simulink model "AERO421_FP6"  (R2024b)
settings: Solver=FixedStepAuto  StartTime=0.0  StopTime=tspan  FixedStep=5  RelTol=1e-5
values from neighbouring files (symbols this model uses):
  E_b_ECI_0 = C2EulerAngles(C_b_ECI_0)    [AERO421_FP6_RJFSR.m]    (also in stefansOldCode.m)
  I_s = diag([1.2, 1.2, 1.2])    [AERO421_FP6_RJFSR.m]    (also in stefansOldCode.m = diag([0.6, 0.6 ,1.2]))
  J = J + I_w1 + I_w2 + I_w3    [AERO421_FP6_RJFSR.m]    (also in stefansOldCode.m = J + I_s)
  Kd = J*eye(3)*2*zeta*wn    [AERO421_FP6_RJFSR.m]    (also in stefansOldCode.m)
  Kp = 2*J*eye(3)*wn^2    [AERO421_FP6_RJFSR.m]    (also in stefansOldCode.m)
  q_b_ECI_0 = rotm2quat(C_b_ECI_0)    [AERO421_FP6_RJFSR.m]    (also in stefansOldCode.m)
  w_b_ECI_0 = [0.001; -0.001; 0.002]    [AERO421_FP6_RJFSR.m]    (also in stefansOldCode.m)
undefined symbols (not defined in the file or in its folder): r_ECI_0, v_ECI_0
libraries: aerolibutil x1
settings Model: Creator=emehiel  LastModifiedBy=rosha
settings SolverCC: AlgebraicLoopSolver=TrustRegion
settings DebuggingCC: UnconnectedInputMsg=warning  UnconnectedOutputMsg=warning  UnconnectedLineMsg=warning
settings ModelReferenceCC: EnableRefExpFcnMdlSchedulingChecks=on
settings RTWCC: GPUComputeCapability=3.5

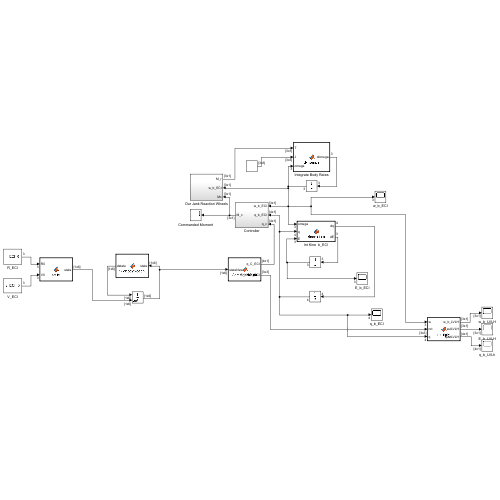
[thumbnail: Simulink's stored preview of the top-level diagram]
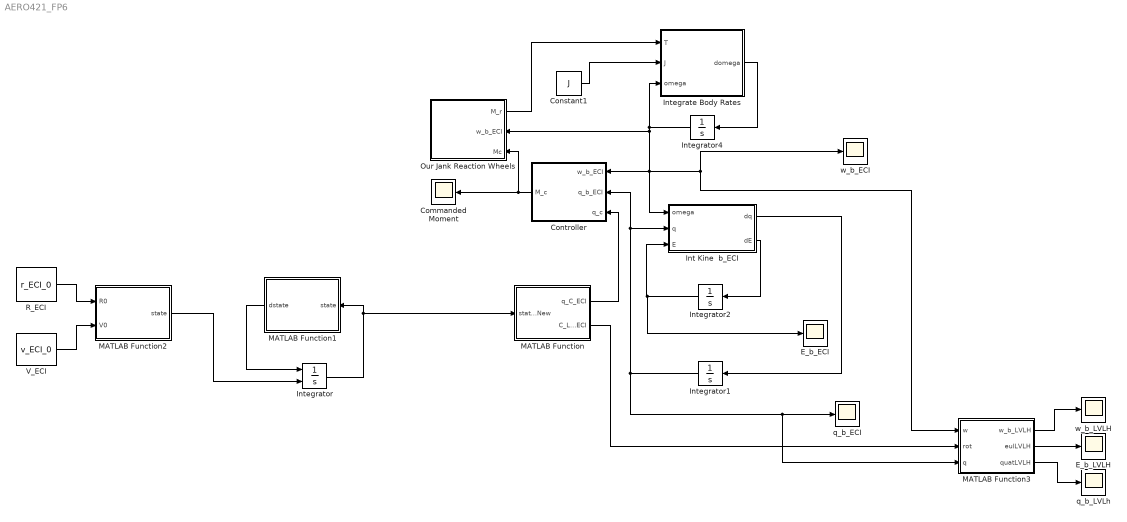
== system AERO421_FP6 ==
  Commanded Moment : Scope
  Constant1 : Constant  Value=J
  Controller : Subsystem
  E_b_ECI : Scope
  E_b_LVLH : Scope
  Int Kine  b_ECI : MATLAB Function  TreatAsAtomicUnit=on
  Integrate Body Rates : MATLAB Function  TreatAsAtomicUnit=on
  Integrator : Integrator  InitialConditionSource=external
  Integrator1 : Integrator  InitialCondition=q_b_ECI_0
  Integrator2 : Integrator  InitialCondition=E_b_ECI_0
  Integrator4 : Integrator  InitialCondition=w_b_ECI_0
  MATLAB Function : MATLAB Function  TreatAsAtomicUnit=on
  MATLAB Function1 : MATLAB Function  TreatAsAtomicUnit=on
  MATLAB Function2 : MATLAB Function  TreatAsAtomicUnit=on
  MATLAB Function3 : MATLAB Function  TreatAsAtomicUnit=on
  Our Jank Reaction Wheels : Subsystem
      settings: PortSchema="{\"entries\":[{\"content\":{\"sides\":[{\"content\":{\"connectorIds\":[\"Out1\",\"In1\",\"In2\"]},\"type\":\"ConnectorPlacement.EquallySpacedRectSide\",\"uuid\":\"c07e65a8-3a09-4163-ab9e-2228d2e52ec5\"},{\"content\":{\"side\":\"RIGHT\"},\"type\":\"ConnectorPlacement.EquallySpacedRectSide\",\"uuid\":\"64fc0568-6df4-40c5-97b1-a675a03b9b7b\"},{\"content\":{\"side\":\"TOP\"},\"type\":\"ConnectorPlacement.EquallySpacedRectSide\",\"uuid\":\"6ced51b5-350f-46bd-bff5-546870cdfb70\"}]},\"type\":\"ConnectorPlacement.EquallySpacedConnector\",\"uuid\":\"a6912720-308f-478a-9475-f02870833daa\"}],\"packageUris\":[\"http://schema.mathworks.com/mf0/Connector/R2020b\"],\"version\":\"1.0\"}"
  R_ECI : Constant  Value=r_ECI_0
  V_ECI : Constant  Value=v_ECI_0
  q_b_ECI : Scope
  q_b_LVLh : Scope
  w_b_ECI : Scope
  w_b_LVLH : Scope
  wires:
  Controller/1(M_c) -> Commanded Moment/1, Our Jank Reaction Wheels/2(Mc)
  Constant1/1 -> Integrate Body Rates/2(J)
  Integrate Body Rates/1(domega) -> Integrator4/1
  Integrator4/1 -> Our Jank Reaction Wheels/1(w_b_ECI), MATLAB Function3/1(w), w_b_ECI/1, Int Kine  b_ECI/1(omega), Controller/1(w_b_ECI), Integrate Body Rates/3(omega)
  Integrator2/1 -> E_b_ECI/1, Int Kine  b_ECI/3(E)
  Integrator1/1 -> Controller/2(q_b_ECI), Int Kine  b_ECI/2(q), MATLAB Function3/3(q), q_b_ECI/1
  Int Kine  b_ECI/2(dE) -> Integrator2/1
  Int Kine  b_ECI/1(dq) -> Integrator1/1
  Our Jank Reaction Wheels/1(M_r) -> Integrate Body Rates/1(T)
  R_ECI/1 -> MATLAB Function2/1(R0)
  V_ECI/1 -> MATLAB Function2/2(V0)
  MATLAB Function/1(q_C_ECI) -> Controller/3(q_c)
  MATLAB Function1/1(dstate) -> Integrator/1
  Integrator/1 -> MATLAB Function/1(stateNew), MATLAB Function1/1(state)
  MATLAB Function2/1(state) -> Integrator/2
  MATLAB Function/2(C_LVLH_ECI) -> MATLAB Function3/2(rot)
  MATLAB Function3/1(w_b_LVLH) -> w_b_LVLH/1
  MATLAB Function3/2(eulLVLH) -> E_b_LVLH/1
  MATLAB Function3/3(quatLVLH) -> q_b_LVLh/1

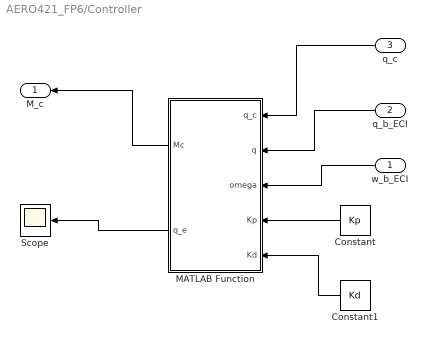
== system AERO421_FP6/Controller ==
  w_b_ECI : Inport  PortDimensions=[3 1]
  q_b_ECI : Inport  Port=2  PortDimensions=[4 1]
  q_c : Inport  Port=3  PortDimensions=[4 1]
  Constant : Constant  Value=Kp
  Constant1 : Constant  Value=Kd
  MATLAB Function : MATLAB Function  TreatAsAtomicUnit=on
  Scope : Scope
  M_c : Outport  PortDimensions=[3 1]  VectorParamsAs1DForOutWhenUnconnected=off
  wires:
  MATLAB Function/1(Mc) -> M_c/1
  q_c/1 -> MATLAB Function/1(q_c)
  q_b_ECI/1 -> MATLAB Function/2(q)
  w_b_ECI/1 -> MATLAB Function/3(omega)
  Constant/1 -> MATLAB Function/4(Kp)
  Constant1/1 -> MATLAB Function/5(Kd)
  MATLAB Function/2(q_e) -> Scope/1

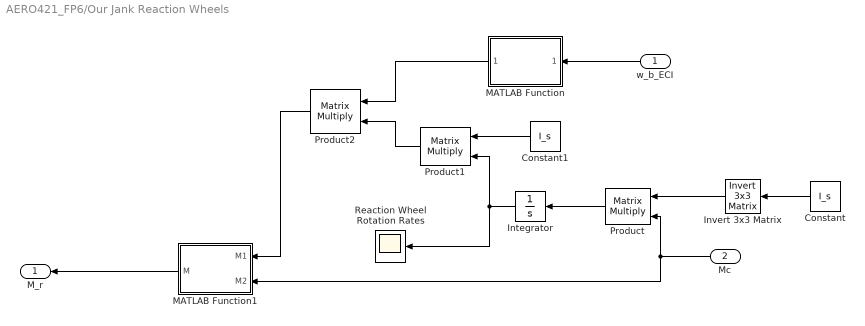
== system AERO421_FP6/Our Jank Reaction Wheels ==
  w_b_ECI : Inport  PortDimensions=[3 1]
  Mc : Inport  Port=2
  Constant : Constant  Value=I_s
  Constant1 : Constant  Value=I_s
  Integrator : Integrator
  Invert 3x3 Matrix : aerolibutil/Invert  3x3 Matrix
  MATLAB Function : MATLAB Function  TreatAsAtomicUnit=on
  MATLAB Function1 : MATLAB Function  TreatAsAtomicUnit=on
  Product : Product  Multiplication=Matrix(*)
  Product1 : Product  Multiplication=Matrix(*)
  Product2 : Product  Multiplication=Matrix(*)
  Reaction Wheel Rotation Rates : Scope
  M_r : Outport  PortDimensions=[3 1]  VectorParamsAs1DForOutWhenUnconnected=off
  wires:
  MATLAB Function1/1(M) -> M_r/1
  Mc/1 -> MATLAB Function1/2(M2), Product/2
  w_b_ECI/1 -> MATLAB Function/1(omega)
  Invert 3x3 Matrix/1 -> Product/1
  Constant/1 -> Invert 3x3 Matrix/1
  Product/1 -> Integrator/1
  Integrator/1 -> Reaction Wheel Rotation Rates/1, Product1/2
  Constant1/1 -> Product1/1
  Product2/1 -> MATLAB Function1/1(M1)
  Product1/1 -> Product2/2
  MATLAB Function/1(omegaX) -> Product2/1

== matlab function AERO421_FP6/Our Jank Reaction Wheels/MATLAB Function1 ==
  data: M1 input; M output; M2 input
function M = matAdd(M1, M2)
M = M1 + M2;

== matlab function AERO421_FP6/Our Jank Reaction Wheels/MATLAB Function ==
  data: omega input; omegaX output
function omegaX = omegaCross(omega)
omegaX = vcross(omega);

== matlab function AERO421_FP6/MATLAB Function ==
  data: stateNew input; q_C_ECI output; C_LVLH_ECI output
function [q_C_ECI,C_LVLH_ECI] = CommandQuat(stateNew)

R = [stateNew(end,1); stateNew(end,2); stateNew(end,3)];
V = [stateNew(end,4); stateNew(end,5); stateNew(end,6)];

R = R'; %in ECI
V = V';

Z_lvlh = -R/norm(R);
Y_lvlh = -cross(R,V)/norm(cross(R,V));
X_lvlh = cross(Y_lvlh,Z_lvlh);

C_LVLH_ECI = [X_lvlh',Y_lvlh',Z_lvlh'];
C_ECI_LVLH = C_LVLH_ECI';

pointingLVLH = [0;0;-1]; %pointing nadir (always at ground station)

eul = C_ECI_LVLH*pointingLVLH;

q = eul2quat(eul')';
n = q(1);
e = q(2:4);

q_C_ECI = [e;n];

== matlab function AERO421_FP6/MATLAB Function1 ==
  data: state input; dstate output
function dstate = twobodymotion(state) %dstate is derivitve of state
%FUNCTION put in descrip    

mu = 398600;

    %define vars
    x = state(1);
    y = state(2);
    z = state(3);
    dx = state(4); %vel
    dy = state(5); %vel
    dz = state(6); %vel
    
    %mag of pos vector
    r = norm([x y z]);
    
    %accel: !!eqs of motion!!
    ddx = -mu*x/r^3;
    ddy = -mu*y/r^3;
    ddz = -mu*z/r^3;
    
    dstate = [dx; dy; dz; ddx; ddy; ddz]';

end

== matlab function AERO421_FP6/Int Kine  b_ECI ==
  data: omega input; q input; dq output; E input; dE output
function [dq,dE] = kinematics(omega, q, E)
%#codegen

% unpack quaternion

epsilon = q(1:3,1);
eta = q(4,1);

depsilon = 1/2*(eta*eye(3) + vcross(epsilon))*omega;
deta = -1/2*epsilon'*omega;

dq = [depsilon; deta];

LBI = 1/cos(E(2))*[cos(E(2)) sin(E(1))*sin(E(2))  cos(E(1))*sin(E(2));
                   0         cos(E(1))*cos(E(2)) -sin(E(1))*cos(E(2));
                   0         sin(E(1))            cos(E(1))];

dE = LBI*omega;

== matlab function AERO421_FP6/Integrate Body Rates ==
  data: T input; J input; omega input; domega output
function domega = dynamics(T, J, omega)
%#codegen

domega = J\(T - cross(omega, J*omega));

== matlab function AERO421_FP6/MATLAB Function2 ==
  data: R0 input; state output; V0 input
function state = state(R0,V0)

state = [R0',V0'];

== matlab function AERO421_FP6/MATLAB Function3 ==
  data: w input; rot input; w_b_LVLH output; q input; eulLVLH output; quatLVLH output
function [w_b_LVLH,eulLVLH,quatLVLH] = multiply(w,rot,q)

w_b_LVLH = rot*w;

n = q(4);
e = q(1:3)';
quat = [n,e];
eul = quat2eul(quat);

eulLVLH = rot*eul';

q2 = eul2quat(eulLVLH')';
n = q2(1);
e = q2(2:4);
quatLVLH = [e;n];

== matlab function AERO421_FP6/Controller/MATLAB Function ==
  data: q_c input; Mc output; q input; omega input; Kp input; Kd input; q_e output
function [Mc,q_e]  = control_law(q_c, q, omega, Kp, Kd)
%#codegen

%q_e = quatMult(quatConjugate(q_c), q);
q_e = quatMult(q, quatConjugate(q_c));
Mc = -Kp*q_e(1:3,1) - Kd*omega;
